simulink model "Week3_problem3"  (R2020b)
settings: Solver=VariableStepAuto  StartTime=0.0  StopTime=25  RelTol=1e-3
InitFcn:
  | Wheel_Slip=0.2;
  | m=75;
  | R=1.25;
  | g=9.81;
  | I=5;
  | v0=44;
  | ABS_CONTROL=1;
undefined symbols (not defined in the file or in its folder): sigbuilder_block
settings Model: Creator=omkar  LastModifiedBy=omkar

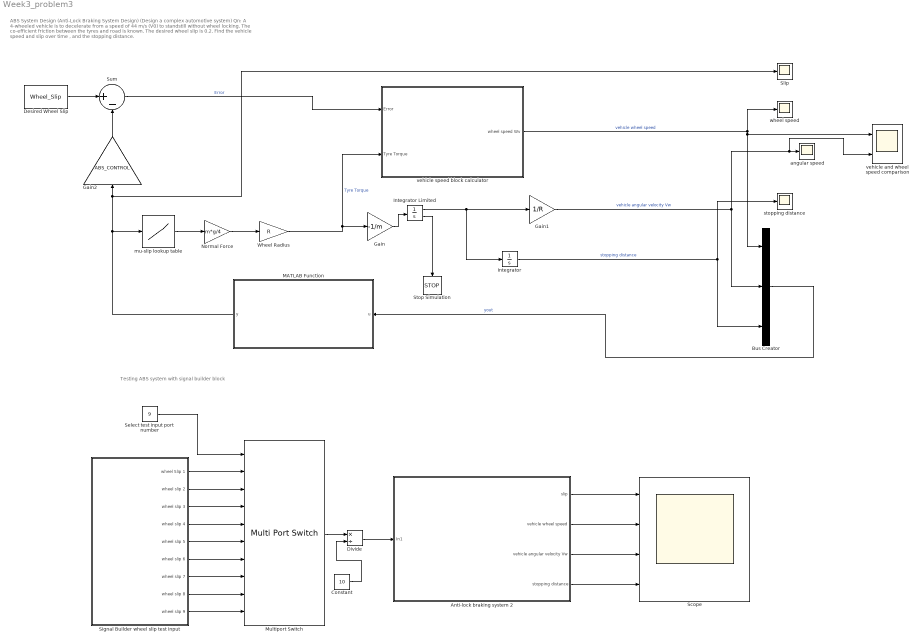
== system Week3_problem3 ==
  note: ABS System Design (Anti-Lock Braking System Design) (Design a complex automotive system)
      | Qn: A 4-wheeled vehicle is to decelerate from a speed of 44 m/s (V0) to standstill without wheel locking. The co-efficient friction between the tyres and road is known. The desired wheel slip is 0.2.
      | Find the vehicle speed and slip over time , and the stopping distance.
  note: Testing ABS system with signal builder block
  Anti-lock braking system 2 : Subsystem
  Bus Creator : BusCreator  Inputs=3
  Constant : Constant  Value=10
  Desired Wheel Slip : Constant  Value=Wheel_Slip
  Divide : Product  Inputs=*/
  Gain : Gain  Gain=-1/m
  Gain1 : Gain  Gain=1/R
  Gain2 : Gain  Gain=ABS_CONTROL
  Integrator : Integrator
  Integrator Limited : Integrator  InitialCondition=v0  LimitOutput=on  UpperSaturationLimit=1000  LowerSaturationLimit=0  ShowSaturationPort=on
  MATLAB Function : MATLAB Function  TreatAsAtomicUnit=on
  Multiport Switch : MultiPortSwitch  Inputs=9  DataPortIndices={2,3,4,5,6,7,8,9,10}  DiagnosticForDefault=None  OutDataTypeStr=int8
  Normal Force : Gain  Gain=m*g/4
  Scope : Scope  NumInputPorts=4
  Select test input port number : Constant  Value=9
  Signal Builder wheel slip test input : Subsystem  Tag=STV Subsys  LoadFcn=sigbuilder_block('load');  StartFcn=sigbuilder_block('start');  StopFcn=sigbuilder_block('stop');  ClipboardFcn=sigbuilder_block('clipboard');  mask(Sigbuilder block){tuvar=[0:10]}
      mask help: Simulink:masks:SigbuilderBlock_MD
      mask init:
      | if ~strcmp(get_param(bdroot(gcbh),'SimulationStatus'),'stopped') tuvar = sigbuilder_block('maskInit'); end
      settings: CopyFcn=sigbuilder_block('copy');  DeleteFcn=sigbuilder_block('delete');  ModelCloseFcn=sigbuilder_block('modelClose');  PreSaveFcn=sigbuilder_block('preSave');  PauseFcn=sigbuilder_block('pause');  ContinueFcn=sigbuilder_block('continue');  NameChangeFcn=sigbuilder_block('namechange');  OpenFcn=sigbuilder_block('open',[5.4 58.2 1141.2 483.6 ]);  CloseFcn=sigbuilder_block('close');
      mask Display: plot(0, 0, 100, 100,[2, 2, 32, 32, 2], [68, 8, 8, 68, 68],[32, 2], [38, 38], [32, 19, 2],[53, 60, 44], [32, 17, 17, 2],[16, 16, 31, 31]);txt = getActiveGroup(gcbh);text(2, 100, txt,'verticalAlignment', 'top');
  Slip : Scope
  Stop Simulation : Stop
  Sum : Sum  Inputs=|+-
  Wheel Radius : Gain  Gain=R
  angular speed : Scope
  mu-slip lookup table : Lookup_n-D  NumberOfTableDimensions=1  BreakpointsForDimension1=|  Table=|  InternalRulePriority=Speed  RndMeth=Simplest  InputSameDT=on
      BreakpointsForDimension1=|
      | [0
      | 0.05
      | 0.1
      | 0.15
      | 0.2
      | 0.25
      | 0.3
      | 0.35
      | 0.4
      | 0.45
      | 0.5
      | 0.55
      | 0.6
      | 0.65
      | 0.7
      | 0.75
      | 0.8
      | 0.85
      | 0.9
      | 0.95
      | 1
      | ]
      Table=|
      | [0
      | 0.4
      | 0.8
      | 0.97
      | 1
      | 0.98
      | 0.96
      | 0.94
      | 0.92
      | 0.9
      | 0.88
      | 0.855
      | 0.83
      | 0.81
      | 0.79
      | 0.77
      | 0.75
      | 0.73
      | 0.72
      | 0.71
      | 0.7
      | ]
  stopping distance : Scope
  vehicle and wheel speed comparison : Scope  NumInputPorts=2
  vehicle speed block calculator : Subsystem
  wheel speed : Scope
  wires:
  Integrator Limited/1 -> Gain1/1, Integrator/1
  Gain1/1 -> vehicle and wheel speed comparison/2, angular speed/1, Bus Creator/2  "vehicle angular velocity Vw"
  Integrator/1 -> stopping distance/1, Bus Creator/3  "stopping distance"
  Integrator Limited/2 -> Stop Simulation/1
  vehicle speed block calculator/1(wheel speed Wv) -> vehicle and wheel speed comparison/1, Bus Creator/1, wheel speed/1  "vehicle wheel speed"
  Sum/1 -> vehicle speed block calculator/1(Error)  "Error"
  Desired Wheel Slip/1 -> Sum/1
  Wheel Radius/1 -> vehicle speed block calculator/2(Tyre Torque), Gain/1  "Tyre Torque"
  mu-slip lookup table/1 -> Normal Force/1
  Gain2/1 -> Sum/2
  Normal Force/1 -> Wheel Radius/1
  Gain/1 -> Integrator Limited/1
  Bus Creator/1 -> MATLAB Function/1(u)  "yout"
  MATLAB Function/1(y) -> mu-slip lookup table/1, Slip/1, Gain2/1
  Anti-lock braking system 2/3(vehicle angular velocity Vw) -> Scope/3
  Anti-lock braking system 2/1(slip) -> Scope/1
  Anti-lock braking system 2/2(vehicle wheel speed) -> Scope/2
  Anti-lock braking system 2/4(stopping distance) -> Scope/4
  Divide/1 -> Anti-lock braking system 2/1(In1)
  Signal Builder wheel slip test input/5(wheel slip 5) -> Multiport Switch/6
  Signal Builder wheel slip test input/1(wheel Slip 1) -> Multiport Switch/2
  Signal Builder wheel slip test input/4(wheel slip 4) -> Multiport Switch/5
  Signal Builder wheel slip test input/2(wheel slip 2) -> Multiport Switch/3
  Signal Builder wheel slip test input/7(wheel slip 7) -> Multiport Switch/8
  Constant/1 -> Divide/2
  Multiport Switch/1 -> Divide/1
  Signal Builder wheel slip test input/9(wheel slip 9) -> Multiport Switch/10
  Signal Builder wheel slip test input/6(wheel slip 6) -> Multiport Switch/7
  Select test input port number/1 -> Multiport Switch/1
  Signal Builder wheel slip test input/3(wheel slip 3) -> Multiport Switch/4
  Signal Builder wheel slip test input/8(wheel slip 8) -> Multiport Switch/9

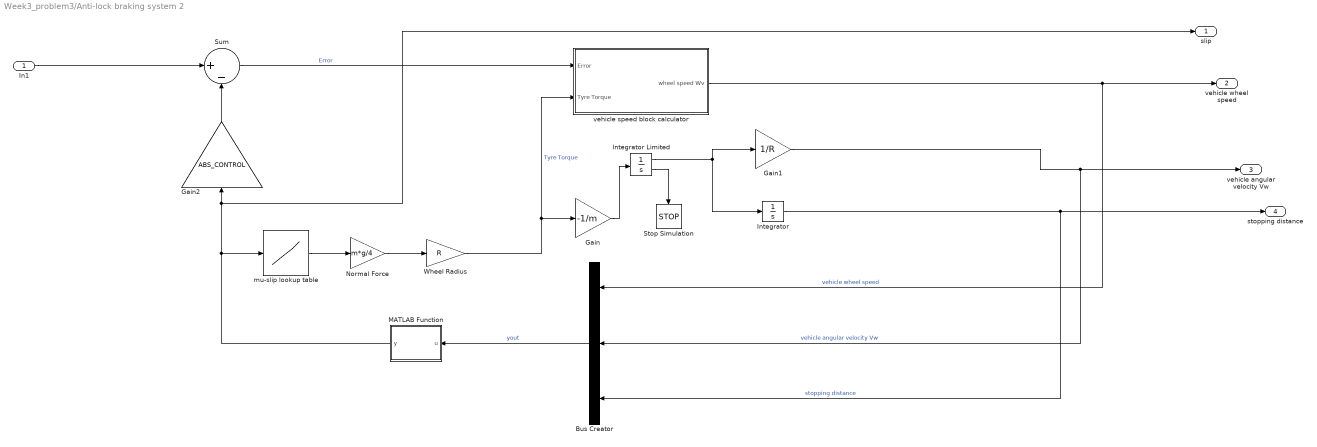
== system Week3_problem3/Anti-lock braking system 2 ==
  In1 : Inport
  Bus Creator : BusCreator  Inputs=3
  Gain : Gain  Gain=-1/m
  Gain1 : Gain  Gain=1/R
  Gain2 : Gain  Gain=ABS_CONTROL
  Integrator : Integrator
  Integrator Limited : Integrator  InitialCondition=v0  LimitOutput=on  UpperSaturationLimit=1000  LowerSaturationLimit=0  ShowSaturationPort=on
  MATLAB Function : MATLAB Function  TreatAsAtomicUnit=on
  Normal Force : Gain  Gain=m*g/4
  Stop Simulation : Stop
  Sum : Sum  Inputs=|+-
  Wheel Radius : Gain  Gain=R
  mu-slip lookup table : Lookup_n-D  NumberOfTableDimensions=1  BreakpointsForDimension1=|  Table=|  InternalRulePriority=Speed  RndMeth=Simplest  InputSameDT=on
      BreakpointsForDimension1=|
      | [0
      | 0.05
      | 0.1
      | 0.15
      | 0.2
      | 0.25
      | 0.3
      | 0.35
      | 0.4
      | 0.45
      | 0.5
      | 0.55
      | 0.6
      | 0.65
      | 0.7
      | 0.75
      | 0.8
      | 0.85
      | 0.9
      | 0.95
      | 1
      | ]
      Table=|
      | [0
      | 0.4
      | 0.8
      | 0.97
      | 1
      | 0.98
      | 0.96
      | 0.94
      | 0.92
      | 0.9
      | 0.88
      | 0.855
      | 0.83
      | 0.81
      | 0.79
      | 0.77
      | 0.75
      | 0.73
      | 0.72
      | 0.71
      | 0.7
      | ]
  vehicle speed block calculator : Subsystem
  slip : Outport
  vehicle wheel speed : Outport  Port=2
  vehicle angular velocity Vw : Outport  Port=3
  stopping distance : Outport  Port=4
  wires:
  Gain/1 -> Integrator Limited/1
  MATLAB Function/1(y) -> mu-slip lookup table/1, slip/1, Gain2/1
  Gain2/1 -> Sum/2
  Gain1/1 -> vehicle angular velocity Vw/1, Bus Creator/2  "vehicle angular velocity Vw"
  Wheel Radius/1 -> vehicle speed block calculator/2(Tyre Torque), Gain/1  "Tyre Torque"
  Normal Force/1 -> Wheel Radius/1
  mu-slip lookup table/1 -> Normal Force/1
  In1/1 -> Sum/1
  Integrator/1 -> stopping distance/1, Bus Creator/3  "stopping distance"
  Bus Creator/1 -> MATLAB Function/1(u)  "yout"
  vehicle speed block calculator/1(wheel speed Wv) -> vehicle wheel speed/1, Bus Creator/1  "vehicle wheel speed"
  Sum/1 -> vehicle speed block calculator/1(Error)  "Error"
  Integrator Limited/2 -> Stop Simulation/1
  Integrator Limited/1 -> Gain1/1, Integrator/1

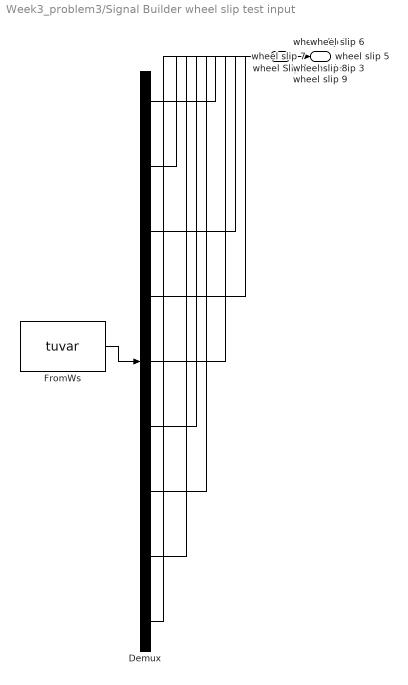
== system Week3_problem3/Signal Builder wheel slip test input ==
  Demux : Demux  Tag=STV Demux  Outputs=9
      settings: DisplayOption=none
  FromWs : FromWorkspace  Tag=STV FromWs  VariableName=tuvar
      SigBuilderData=|
      | common.afterFinalStr = 'Extrapolate'
      | common.sampleTime = 0
      | dataSet.timeRange = [0 10]
      | dataSet.name = 'Group 1'
      | sbobj.Groups.Name = 'Group 1'
      | sbobj.Groups.Signals(1).Name = 'wheel Slip 1'
      | sbobj.Groups.Signals(1).XData = [0 10]
      | sbobj.Groups.Signals(1).YData = [2 2]
      | sbobj.Groups.Signals(2).Name = 'wheel slip 2'
      | sbobj.Groups.Signals(2).XData = [0 10]
      | sbobj.Groups.Signals(2).YData = [3 3]
      | sbobj.Groups.Signals(3).Name = 'wheel slip 3'
      | sbobj.Groups.Signals(3).XData = [0 10]
      | sbobj.Groups.Signals(3).YData = [4 4]
      | sbobj.Groups.Signals(4).Name = 'wheel slip 4'
      | sbobj.Groups.Signals(4).XData = [0 10]
      | sbobj.Groups.Signals(4).YData = [5 5]
      | sbobj.Groups.Signals(5).Name = 'wheel slip 5'
      | sbobj.Groups.Signals(5).XData = [0 10]
      | sbobj.Groups.Signals(5).YData = [6 6]
      | sbobj.Groups.Signals(6).Name = 'wheel slip 6'
      | sbobj.Groups.Signals(6).XData = [0 10]
      | sbobj.Groups.Signals(6).YData = [7 7]
      | sbobj.Groups.Signals(7).Name = 'wheel slip 7'
      | sbobj.Groups.Signals(7).XData = [0 10]
      | sbobj.Groups.Signals(7).YData = [8 8]
      | sbobj.Groups.Signals(8).Name = 'wheel slip 8'
      | sbobj.Groups.Signals(8).XData = [0 10]
      | sbobj.Groups.Signals(8).YData = [9 9]
      | sbobj.Groups.Signals(9).Name = 'wheel slip 9'
      | sbobj.Groups.Signals(9).XData = [0 10]
      | sbobj.Groups.Signals(9).YData = [10 10]
  wheel Slip 1 : Outport  Tag=STV Outport
  wheel slip 2 : Outport  Tag=STV Outport  Port=2
  wheel slip 3 : Outport  Tag=STV Outport  Port=3
  wheel slip 4 : Outport  Tag=STV Outport  Port=4
  wheel slip 5 : Outport  Tag=STV Outport  Port=5
  wheel slip 6 : Outport  Tag=STV Outport  Port=6
  wheel slip 7 : Outport  Tag=STV Outport  Port=7
  wheel slip 8 : Outport  Tag=STV Outport  Port=8
  wheel slip 9 : Outport  Tag=STV Outport  Port=9
  wires:
  FromWs/1 -> Demux/1
  Demux/1 -> wheel Slip 1/1
  Demux/2 -> wheel slip 2/1
  Demux/3 -> wheel slip 3/1
  Demux/4 -> wheel slip 4/1
  Demux/5 -> wheel slip 5/1
  Demux/6 -> wheel slip 6/1
  Demux/7 -> wheel slip 7/1
  Demux/8 -> wheel slip 8/1
  Demux/9 -> wheel slip 9/1

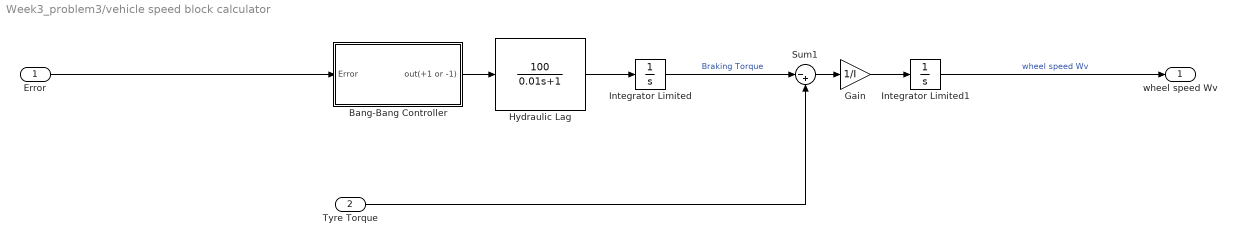
== system Week3_problem3/vehicle speed block calculator ==
  Error : Inport
  Tyre Torque : Inport  Port=2
  Bang-Bang Controller : Subsystem
  Gain : Gain  Gain=1/I
  Hydraulic Lag : TransferFcn  Numerator=[100]  Denominator=[0.01 1]
  Integrator Limited : Integrator  LimitOutput=on  UpperSaturationLimit=1000  LowerSaturationLimit=0
  Integrator Limited1 : Integrator  InitialCondition=v0/R  LimitOutput=on  UpperSaturationLimit=1000  LowerSaturationLimit=0
  Sum1 : Sum  Inputs=|-+
  wheel speed Wv : Outport
  wires:
  Integrator Limited1/1 -> wheel speed Wv/1  "wheel speed Wv"
  Integrator Limited/1 -> Sum1/1  "Braking Torque"
  Gain/1 -> Integrator Limited1/1
  Bang-Bang Controller/1(out(+1 or -1)) -> Hydraulic Lag/1
  Hydraulic Lag/1 -> Integrator Limited/1
  Error/1 -> Bang-Bang Controller/1(Error)
  Tyre Torque/1 -> Sum1/2
  Sum1/1 -> Gain/1

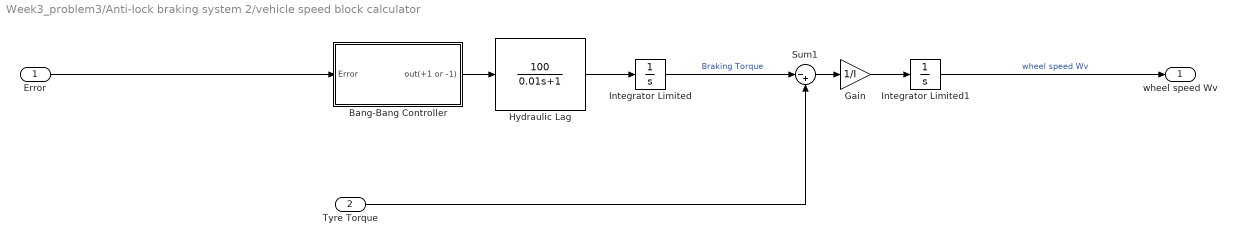
== system Week3_problem3/Anti-lock braking system 2/vehicle speed block calculator ==
  Error : Inport
  Tyre Torque : Inport  Port=2
  Bang-Bang Controller : Subsystem
  Gain : Gain  Gain=1/I
  Hydraulic Lag : TransferFcn  Numerator=[100]  Denominator=[0.01 1]
  Integrator Limited : Integrator  LimitOutput=on  UpperSaturationLimit=1000  LowerSaturationLimit=0
  Integrator Limited1 : Integrator  InitialCondition=v0/R  LimitOutput=on  UpperSaturationLimit=1000  LowerSaturationLimit=0
  Sum1 : Sum  Inputs=|-+
  wheel speed Wv : Outport
  wires:
  Integrator Limited1/1 -> wheel speed Wv/1  "wheel speed Wv"
  Integrator Limited/1 -> Sum1/1  "Braking Torque"
  Gain/1 -> Integrator Limited1/1
  Bang-Bang Controller/1(out(+1 or -1)) -> Hydraulic Lag/1
  Hydraulic Lag/1 -> Integrator Limited/1
  Error/1 -> Bang-Bang Controller/1(Error)
  Tyre Torque/1 -> Sum1/2
  Sum1/1 -> Gain/1

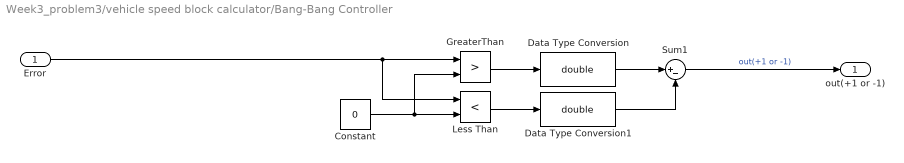
== system Week3_problem3/vehicle speed block calculator/Bang-Bang Controller ==
  Error : Inport
  Constant : Constant  Value=0
  Data Type Conversion : DataTypeConversion  OutDataTypeStr=double  RndMeth=Zero
  Data Type Conversion1 : DataTypeConversion  OutDataTypeStr=double  RndMeth=Zero
  GreaterThan : RelationalOperator  Operator=>  OutDataTypeStr=boolean  RndMeth=Simplest
  Less Than : RelationalOperator  Operator=<  OutDataTypeStr=boolean  RndMeth=Simplest
  Sum1 : Sum  Inputs=|+-
  out(+1 or -1) : Outport
  wires:
  GreaterThan/1 -> Data Type Conversion/1
  Sum1/1 -> out(+1 or -1)/1  "out(+1 or -1)"
  Error/1 -> Less Than/1, GreaterThan/1
  Constant/1 -> GreaterThan/2, Less Than/2
  Data Type Conversion/1 -> Sum1/1
  Data Type Conversion1/1 -> Sum1/2
  Less Than/1 -> Data Type Conversion1/1

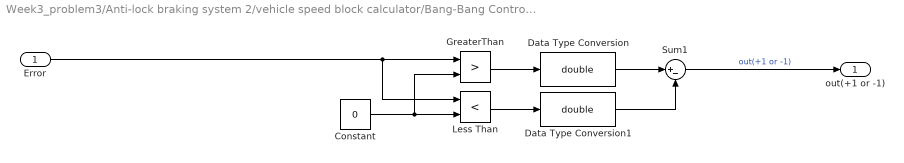
== system Week3_problem3/Anti-lock braking system 2/vehicle speed block calculator/Bang-Bang Controller ==
  Error : Inport
  Constant : Constant  Value=0
  Data Type Conversion : DataTypeConversion  OutDataTypeStr=double  RndMeth=Zero
  Data Type Conversion1 : DataTypeConversion  OutDataTypeStr=double  RndMeth=Zero
  GreaterThan : RelationalOperator  Operator=>  OutDataTypeStr=boolean  RndMeth=Simplest
  Less Than : RelationalOperator  Operator=<  OutDataTypeStr=boolean  RndMeth=Simplest
  Sum1 : Sum  Inputs=|+-
  out(+1 or -1) : Outport
  wires:
  GreaterThan/1 -> Data Type Conversion/1
  Sum1/1 -> out(+1 or -1)/1  "out(+1 or -1)"
  Error/1 -> Less Than/1, GreaterThan/1
  Constant/1 -> GreaterThan/2, Less Than/2
  Data Type Conversion/1 -> Sum1/1
  Data Type Conversion1/1 -> Sum1/2
  Less Than/1 -> Data Type Conversion1/1

== matlab function Week3_problem3/MATLAB Function ==
  data: u input; y output
function y = RelativeSlip(u)
y=1.0 - u(1)/(u(2) + (u(2)==0)*eps);

== matlab function Week3_problem3/Anti-lock braking system 2/MATLAB Function ==
  data: u input; y output
function y = RelativeSlip(u)
y=1.0 - u(1)/(u(2) + (u(2)==0)*eps);
